simulink model "tallercontrol"  (R2022b)
settings: Solver=VariableStepAuto  StartTime=0.0  StopTime=400  RelTol=1e-3
settings Model: Creator=Jhonatan  LastModifiedBy=Jhonatan

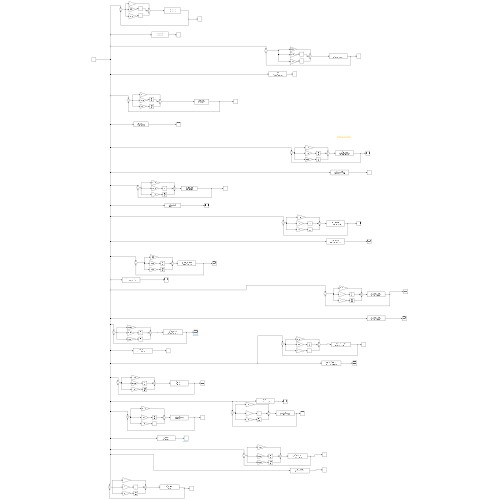
[thumbnail: Simulink's stored preview of the top-level diagram]
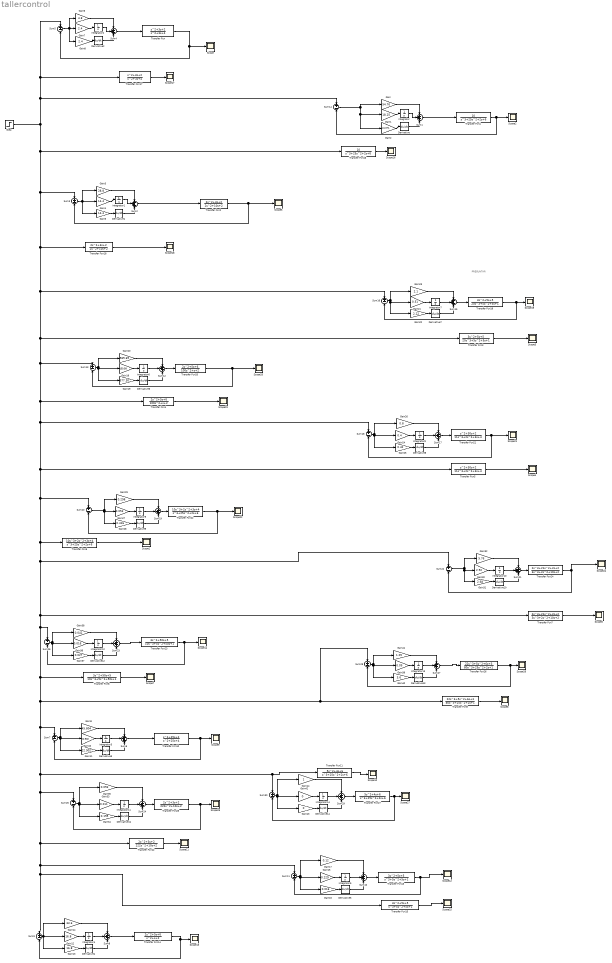
== system tallercontrol ==
  note: PREGUNTAR
  Derivative{,1..14} (15 alike) : Derivative
  Gain : Gain  Gain=54.76
  Gain1 : Gain  Gain=18.25
  Gain10 : Gain  Gain=22.902
  Gain11 : Gain  Gain=22.902
  Gain12 : Gain  Gain=16.8
  Gain13 : Gain  Gain=16.8
  Gain14 : Gain  Gain=33.6
  Gain15 : Gain  Gain=0.229
  Gain16 : Gain  Gain=0.016
  Gain17 : Gain  Gain=0.12
  Gain18 : Gain  Gain=150.58
  Gain19 : Gain  Gain=577.30
  Gain2 : Gain  Gain=41.071
  Gain20 : Gain  Gain=589.69
  Gain21 : Gain  Gain=0.51
  Gain22 : Gain  Gain=2.22
  Gain23 : Gain  Gain=2.1
  Gain24 : Gain  Gain=0.4
  Gain25 : Gain  Gain=0.42
  Gain26 : Gain  Gain=0.8
  Gain27 : Gain  Gain=0.053
  Gain28 : Gain  Gain=0.416
  Gain29 : Gain  Gain=0.298
  Gain3 : Gain  Gain=28.8
  Gain30 : Gain  Gain=2.92
  Gain31 : Gain  Gain=2.68
  Gain32 : Gain  Gain=5.76
  Gain33 : Gain  Gain=0.011
  Gain34 : Gain  Gain=0.195
  Gain35 : Gain  Gain=0.093
  Gain36 : Gain  Gain=0.016
  Gain37 : Gain  Gain=0.027
  Gain38 : Gain  Gain=0.042
  Gain39 : Gain  Gain=0.09
  Gain4 : Gain  Gain=14.4
  Gain40 : Gain  Gain=3.6
  Gain41 : Gain  Gain=1.05
  Gain42 : Gain  Gain=0
  Gain43 : Gain  Gain=0
  Gain44 : Gain
  Gain5 : Gain  Gain=14.4
  Gain6 : Gain  Gain=4.8
  Gain7 : Gain  Gain=2.4
  Gain8 : Gain  Gain=2.4
  Gain9 : Gain  Gain=45.804
  Integrator{,1..14} (15 alike) : Integrator
  Scope{,1..27} (28 alike) : Scope
  Step : Step  SampleTime=0
  Sum{1..2,4,6,8,10,12,15,17,19,21,23..24,27,29} (15 alike) : Sum  Inputs=+++
  Sum{3,5,7,9,11,13..14,16,18,20,22,25..26,28,30} (15 alike) : Sum  Inputs=+-
  Transfer Fcn : TransferFcn  Numerator=[1 3 2]  Denominator=[1 3 4]
  Transfer Fcn1 : TransferFcn  Numerator=[10]  Denominator=[1 25 2 6]
  Transfer Fcn10 : TransferFcn  Numerator=[1 25 2]  Denominator=[1 25 4]
  Transfer Fcn11 : TransferFcn  Numerator=[5 4 6]  Denominator=[1 25 2 6]
  Transfer Fcn12 : TransferFcn  Numerator=[2 3 2]  Denominator=[222 10 2]
  Transfer Fcn13 : TransferFcn  Numerator=[3 5 5]  Denominator=[1 5 5 1]
  Transfer Fcn14 : TransferFcn  Numerator=[2 5 6]  Denominator=[1 1 2]
  Transfer Fcn15 : TransferFcn  Numerator=[3 5 5]  Denominator=[1 5 5 1]
  Transfer Fcn16 : TransferFcn  Numerator=[10]  Denominator=[1 25 2 6]
  Transfer Fcn17 : TransferFcn  Numerator=[1 3 2]  Denominator=[1 3 4]
  Transfer Fcn18 : TransferFcn  Numerator=[2 3 2]  Denominator=[2 10 2]
  Transfer Fcn19 : TransferFcn  Numerator=[3 5 5]  Denominator=[20 5 5 1]
  Transfer Fcn2 : TransferFcn  Numerator=[2 3 2]  Denominator=[2 10 2]
  Transfer Fcn20 : TransferFcn  Numerator=[2 5 6]  Denominator=[100 1 2]
  Transfer Fcn21 : TransferFcn  Numerator=[1 30 2]  Denominator=[11 2 3 4]
  Transfer Fcn22 : TransferFcn  Numerator=[10 2 3 4]  Denominator=[1 25 2 6]
  Transfer Fcn23 : TransferFcn  Numerator=[3 50 5]  Denominator=[10 5 50 1]
  Transfer Fcn24 : TransferFcn  Numerator=[2 21 2 2]  Denominator=[3 2 10 2]
  Transfer Fcn25 : TransferFcn  Numerator=[2 3 2]  Denominator=[222 10 2]
  Transfer Fcn26 : TransferFcn  Numerator=[22 5 6 3]  Denominator=[80 25 2 1]
  Transfer Fcn27 : TransferFcn  Numerator=[5 4 6]  Denominator=[1 25 2 6]
  Transfer Fcn3 : TransferFcn  Numerator=[3 5 5]  Denominator=[20 5 5 1]
  Transfer Fcn4 : TransferFcn  Numerator=[2 5 6]  Denominator=[100 1 2]
  Transfer Fcn5 : TransferFcn  Numerator=[1 30 2]  Denominator=[11 2 3 4]
  Transfer Fcn6 : TransferFcn  Numerator=[10 2 3 4]  Denominator=[1 25 2 6]
  Transfer Fcn7 : TransferFcn  Numerator=[2 21 2 2]  Denominator=[3 2 10 2]
  Transfer Fcn8 : TransferFcn  Numerator=[3 50 5]  Denominator=[10 5 50 1]
  Transfer Fcn9 : TransferFcn  Numerator=[22 5 6 3]  Denominator=[80 25 2 1]
  wires:
  Transfer Fcn/1 -> Sum5/2, Scope/1
  Transfer Fcn1/1 -> Scope2/1, Sum14/2
  Transfer Fcn2/1 -> Sum3/2, Scope5/1
  Transfer Fcn3/1 -> Scope3/1
  Transfer Fcn4/1 -> Scope23/1
  Gain1/1 -> Integrator/1
  Gain2/1 -> Derivative/1
  Derivative/1 -> Sum1/3
  Integrator/1 -> Sum1/2
  Gain/1 -> Sum1/1
  Transfer Fcn6/1 -> Scope1/1
  Transfer Fcn8/1 -> Scope7/1
  Transfer Fcn9/1 -> Scope8/1
  Transfer Fcn10/1 -> Sum7/2, Scope9/1
  Transfer Fcn11/1 -> Scope10/1
  Transfer Fcn12/1 -> Scope11/1
  Transfer Fcn14/1 -> Sum9/2, Scope13/1
  Gain4/1 -> Integrator1/1
  Gain3/1 -> Sum2/1
  Derivative1/1 -> Sum2/3
  Sum3/1 -> Gain4/1, Gain5/1, Gain3/1
  Gain5/1 -> Derivative1/1
  Integrator1/1 -> Sum2/2
  Gain7/1 -> Integrator2/1
  Gain6/1 -> Sum4/1
  Derivative2/1 -> Sum4/3
  Sum4/1 -> Transfer Fcn/1
  Gain8/1 -> Derivative2/1
  Integrator2/1 -> Sum4/2
  Sum5/1 -> Gain8/1, Gain7/1, Gain6/1
  Sum2/1 -> Transfer Fcn2/1
  Gain11/1 -> Derivative3/1
  Integrator3/1 -> Sum6/2
  Gain10/1 -> Integrator3/1
  Derivative3/1 -> Sum6/3
  Sum7/1 -> Gain10/1, Gain11/1, Gain9/1
  Gain9/1 -> Sum6/1
  Sum6/1 -> Transfer Fcn10/1
  Transfer Fcn13/1 -> Scope12/1, Sum11/2
  Sum9/1 -> Gain14/1, Gain12/1, Gain13/1
  Gain14/1 -> Sum8/1
  Derivative4/1 -> Sum8/3
  Gain12/1 -> Integrator4/1
  Integrator4/1 -> Sum8/2
  Gain13/1 -> Derivative4/1
  Sum8/1 -> Transfer Fcn14/1
  Sum11/1 -> Gain15/1, Gain16/1, Gain17/1
  Gain17/1 -> Sum10/1
  Derivative5/1 -> Sum10/3
  Gain15/1 -> Integrator5/1
  Integrator5/1 -> Sum10/2
  Gain16/1 -> Derivative5/1
  Sum10/1 -> Transfer Fcn13/1
  Sum1/1 -> Transfer Fcn1/1
  Sum14/1 -> Gain2/1, Gain1/1, Gain/1
  Transfer Fcn15/1 -> Scope15/1
  Transfer Fcn16/1 -> Scope16/1
  Transfer Fcn17/1 -> Scope17/1
  Transfer Fcn18/1 -> Scope18/1
  Gain22/1 -> Derivative7/1
  Integrator7/1 -> Sum15/2
  Gain21/1 -> Integrator7/1
  Derivative7/1 -> Sum15/3
  Gain23/1 -> Sum15/1
  Sum15/1 -> Transfer Fcn19/1
  Sum16/1 -> Gain21/1, Gain22/1, Gain23/1
  Transfer Fcn19/1 -> Scope19/1, Sum16/2
  Transfer Fcn20/1 -> Sum13/2, Scope20/1
  Sum12/1 -> Transfer Fcn20/1
  Gain20/1 -> Sum12/1
  Derivative6/1 -> Sum12/3
  Sum13/1 -> Gain18/1, Gain19/1, Gain20/1
  Gain18/1 -> Integrator6/1
  Integrator6/1 -> Sum12/2
  Gain19/1 -> Derivative6/1
  Derivative8/1 -> Sum17/3
  Gain26/1 -> Sum17/1
  Sum17/1 -> Transfer Fcn21/1
  Gain25/1 -> Derivative8/1
  Integrator8/1 -> Sum17/2
  Gain24/1 -> Integrator8/1
  Sum18/1 -> Gain24/1, Gain25/1, Gain26/1
  Transfer Fcn21/1 -> Scope21/1, Sum18/2
  Transfer Fcn22/1 -> Sum20/2, Scope22/1
  Derivative9/1 -> Sum19/3
  Gain29/1 -> Sum19/1
  Gain28/1 -> Derivative9/1
  Sum20/1 -> Gain27/1, Gain28/1, Gain29/1
  Integrator9/1 -> Sum19/2
  Gain27/1 -> Integrator9/1
  Sum19/1 -> Transfer Fcn22/1
  Transfer Fcn24/1 -> Sum22/2, Scope24/1
  Derivative10/1 -> Sum21/3
  Gain32/1 -> Sum21/1
  Sum22/1 -> Gain30/1, Gain31/1, Gain32/1
  Integrator10/1 -> Sum21/2
  Sum21/1 -> Transfer Fcn24/1
  Gain31/1 -> Derivative10/1
  Gain30/1 -> Integrator10/1
  Transfer Fcn7/1 -> Scope6/1
  Transfer Fcn5/1 -> Scope4/1
  Sum25/1 -> Gain33/1, Gain34/1, Gain35/1
  Derivative11/1 -> Sum24/3
  Gain34/1 -> Derivative11/1
  Gain35/1 -> Sum24/1
  Integrator11/1 -> Sum24/2
  Transfer Fcn25/1 -> Sum25/2, Scope25/1
  Gain33/1 -> Integrator11/1
  Sum24/1 -> Transfer Fcn25/1
  Gain38/1 -> Sum23/1
  Derivative12/1 -> Sum23/3
  Integrator12/1 -> Sum23/2
  Transfer Fcn23/1 -> Sum26/2, Scope14/1
  Gain36/1 -> Integrator12/1
  Sum26/1 -> Gain36/1, Gain37/1, Gain38/1
  Gain37/1 -> Derivative12/1
  Sum23/1 -> Transfer Fcn23/1
  Sum28/1 -> Gain39/1, Gain40/1, Gain41/1
  Gain40/1 -> Derivative13/1
  Integrator13/1 -> Sum27/2
  Gain39/1 -> Integrator13/1
  Transfer Fcn26/1 -> Sum28/2, Scope26/1
  Sum27/1 -> Transfer Fcn26/1
  Derivative13/1 -> Sum27/3
  Gain41/1 -> Sum27/1
  Step/1 -> Transfer Fcn16/1, Sum3/1, Transfer Fcn18/1, Sum16/1, Sum13/1, Transfer Fcn4/1, Sum18/1, Sum20/1, Transfer Fcn6/1, Sum22/1, Sum26/1, Sum7/1, Sum25/1, Transfer Fcn12/1, Transfer Fcn15/1, Sum9/1, Sum11/1, Sum30/1, Transfer Fcn11/1, Sum28/1, Transfer Fcn9/1, Transfer Fcn8/1, Transfer Fcn7/1, Transfer Fcn5/1, Transfer Fcn3/1, Sum5/1, Transfer Fcn17/1, Sum14/1
  Derivative14/1 -> Sum29/3
  Gain42/1 -> Integrator14/1
  Sum29/1 -> Transfer Fcn27/1
  Sum30/1 -> Gain42/1, Gain43/1, Gain44/1
  Gain44/1 -> Sum29/1
  Gain43/1 -> Derivative14/1
  Integrator14/1 -> Sum29/2
  Transfer Fcn27/1 -> Sum30/2, Scope27/1
